simulink model "ssModl"  (R2024a)
settings: Solver=VariableStepAuto  StartTime=0.0  StopTime=10.0  RelTol=1e-3
settings Model: Creator=farza  LastModifiedBy=farza

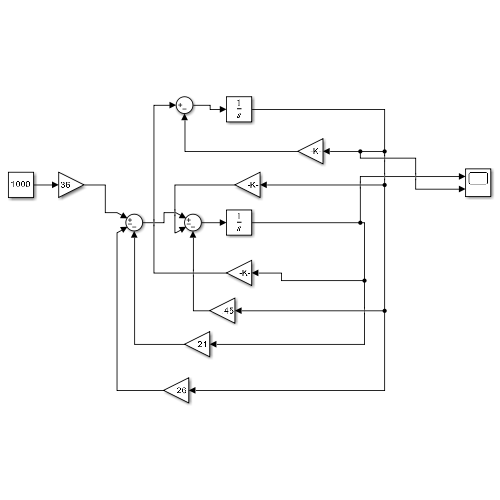
[thumbnail: Simulink's stored preview of the top-level diagram]
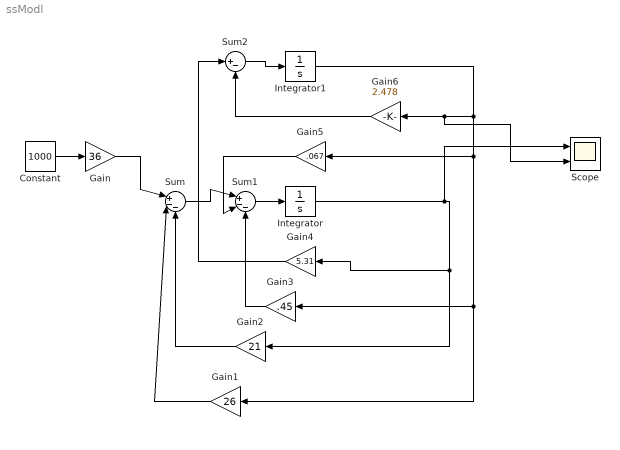
== system ssModl ==
  Constant : Constant  Value=1000
  Gain : Gain  Gain=36
  Gain1 : Gain  Gain=26
  Gain2 : Gain  Gain=21
  Gain3 : Gain  Gain=.45
  Gain4 : Gain  Gain=5.31
  Gain5 : Gain  Gain=.067
  Gain6 : Gain  Gain=2.478
  Integrator : Integrator
  Integrator1 : Integrator
  Scope : Scope  NumInputPorts=2
  Sum : Sum  Inputs=|+--
  Sum1 : Sum  Inputs=|+--
  Sum2 : Sum  Inputs=|+-
  wires:
  Constant/1 -> Gain/1
  Gain/1 -> Sum/1
  Gain1/1 -> Sum/2
  Gain2/1 -> Sum/3
  Sum/1 -> Sum1/1
  Gain3/1 -> Sum1/3
  Sum1/1 -> Integrator/1
  Integrator/1 -> Scope/1, Gain4/1, Gain2/1
  Gain5/1 -> Sum1/2
  Sum2/1 -> Integrator1/1
  Gain4/1 -> Sum2/1
  Gain6/1 -> Sum2/2
  Integrator1/1 -> Gain1/1, Gain3/1, Gain5/1, Scope/2, Gain6/1
